simulink model "main_damaged_aircraft"  (R2025b)
settings: Solver=ode45  StartTime=0.0  StopTime=10  RelTol=1e-3
InitFcn:
  | init_project;
undefined symbols (not defined in the file): P, theta_d
libraries: aerolibprivatev1p5 x2, aerolibatmos2 x1, aerolibobsolete x1
settings Model: Creator=22149  LastModifiedBy=22149
settings DataIOCC: SaveFormat=StructureWithTime

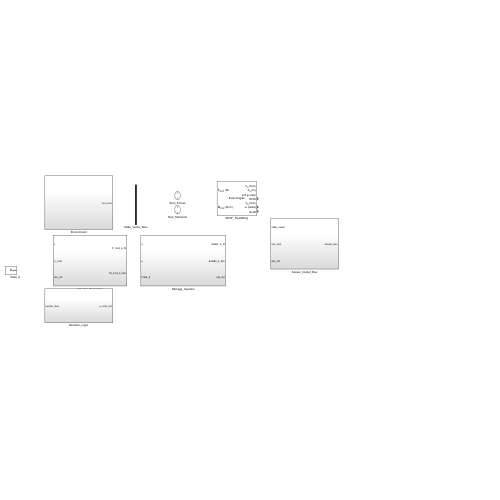
[thumbnail: Simulink's stored preview of the top-level diagram]
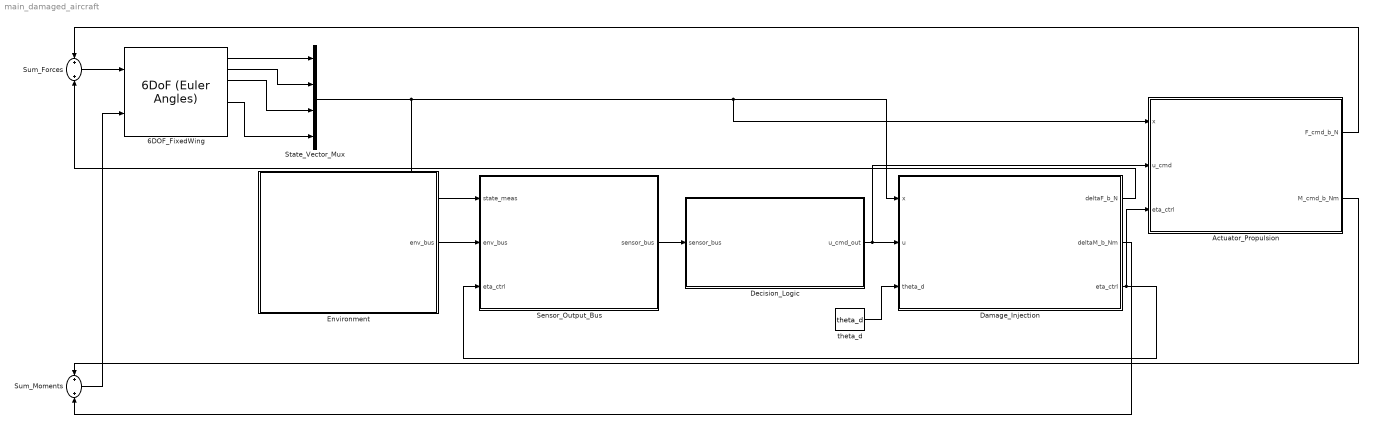
== system main_damaged_aircraft ==
  6DOF_FixedWing : aerolibprivatev1p5/6DoF (Euler Angles)  xme_0=P.initial.pned_m'  Vm_0=P.initial.uvw_mps'  eul_0=P.initial.euler_rad'  pm_0=P.initial.pqr_rps'  Mass=P.aircraft.mass  Inertia=P.aircraft.inertia
  Actuator_Propulsion : Subsystem
  Damage_Injection : Subsystem
  Decision_Logic : Subsystem
  Environment : Subsystem
  Sensor_Output_Bus : Subsystem
  State_Vector_Mux : Mux
  Sum_Forces : Sum
  Sum_Moments : Sum
  theta_d : Constant  Value=theta_d
  wires:
  Sum_Forces/1 -> 6DOF_FixedWing/1
  Sensor_Output_Bus/1(sensor_bus) -> Decision_Logic/1(sensor_bus)
  6DOF_FixedWing/2 -> State_Vector_Mux/2
  Sum_Moments/1 -> 6DOF_FixedWing/2
  theta_d/1 -> Damage_Injection/3(theta_d)
  6DOF_FixedWing/1 -> State_Vector_Mux/1
  6DOF_FixedWing/3 -> State_Vector_Mux/3
  State_Vector_Mux/1 -> Actuator_Propulsion/1(x), Damage_Injection/1(x), Sensor_Output_Bus/1(state_meas)
  Environment/1(env_bus) -> Sensor_Output_Bus/2(env_bus)
  6DOF_FixedWing/5 -> State_Vector_Mux/4
  Decision_Logic/1(u_cmd_out) -> Actuator_Propulsion/2(u_cmd), Damage_Injection/2(u)
  Damage_Injection/1(deltaF_b_N) -> Sum_Forces/2
  Damage_Injection/2(deltaM_b_Nm) -> Sum_Moments/2
  Damage_Injection/3(eta_ctrl) -> Sensor_Output_Bus/3(eta_ctrl), Actuator_Propulsion/3(eta_ctrl)
  Actuator_Propulsion/1(F_cmd_b_N) -> Sum_Forces/1
  Actuator_Propulsion/2(M_cmd_b_Nm) -> Sum_Moments/1

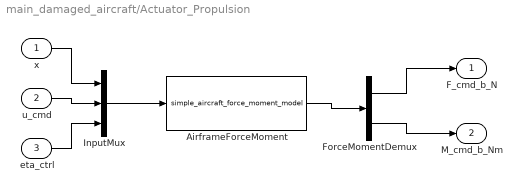
== system main_damaged_aircraft/Actuator_Propulsion ==
  x : Inport
  u_cmd : Inport  Port=2
  eta_ctrl : Inport  Port=3
  AirframeForceMoment : MATLABFcn  MATLABFcn=simple_aircraft_force_moment_model  OutputDimensions=6
  ForceMomentDemux : Demux  Outputs=[3 3]
  InputMux : Mux  Inputs=3
  F_cmd_b_N : Outport
  M_cmd_b_Nm : Outport  Port=2
  wires:
  x/1 -> InputMux/1
  u_cmd/1 -> InputMux/2
  eta_ctrl/1 -> InputMux/3
  InputMux/1 -> AirframeForceMoment/1
  AirframeForceMoment/1 -> ForceMomentDemux/1
  ForceMomentDemux/1 -> F_cmd_b_N/1
  ForceMomentDemux/2 -> M_cmd_b_Nm/1

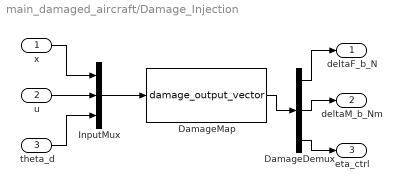
== system main_damaged_aircraft/Damage_Injection ==
  x : Inport
  u : Inport  Port=2
  theta_d : Inport  Port=3
  DamageDemux : Demux  Outputs=[3 3 4]
  DamageMap : MATLABFcn  MATLABFcn=damage_output_vector  OutputDimensions=10
  InputMux : Mux  Inputs=3
  deltaF_b_N : Outport
  deltaM_b_Nm : Outport  Port=2
  eta_ctrl : Outport  Port=3
  wires:
  x/1 -> InputMux/1
  u/1 -> InputMux/2
  theta_d/1 -> InputMux/3
  InputMux/1 -> DamageMap/1
  DamageMap/1 -> DamageDemux/1
  DamageDemux/1 -> deltaF_b_N/1
  DamageDemux/2 -> deltaM_b_Nm/1
  DamageDemux/3 -> eta_ctrl/1

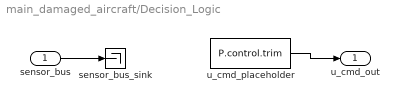
== system main_damaged_aircraft/Decision_Logic ==
  sensor_bus : Inport
  sensor_bus_sink : Terminator
  u_cmd_placeholder : Constant  Value=P.control.trim
  u_cmd_out : Outport
  wires:
  sensor_bus/1 -> sensor_bus_sink/1
  u_cmd_placeholder/1 -> u_cmd_out/1

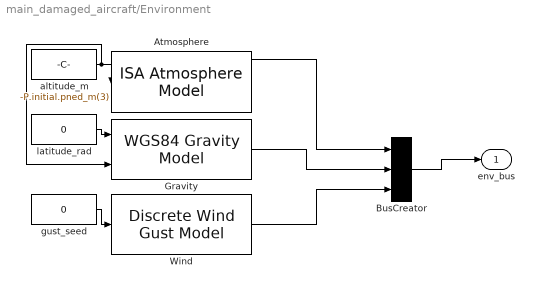
== system main_damaged_aircraft/Environment ==
  Atmosphere : aerolibatmos2/ISA Atmosphere Model  useExtended=off  action=None  custom=off  viscosityOut=off  g=9.80665  gamma=1.4  R=287.0531  L=0.0065  h_trop=11000  h_strat=20000  rho0=1.225  P0=101325  T0=288.15  h0=0  S=110.4  Tref=273.15  muref=1.716e-5
  BusCreator : BusCreator  Inputs=3
  Gravity : aerolibobsolete/WGS84 Gravity Model  model=WGS84 Taylor Series  units=Metric (MKS)  no_atmos=on  precessing=on  month=February  day=1  year=2000  no_centrifugal=on  action=Warning
  Wind : aerolibprivatev1p5/Discrete Wind Gust Model  v_units=meters/second  Gx=on  Gy=on  Gz=on  t_0=5  d_m=[120 120 80]  v_m=[3.5 3.5 3.0]
  altitude_m : Constant  Value=-P.initial.pned_m(3)
  gust_seed : Constant  Value=0
  latitude_rad : Constant  Value=0
  env_bus : Outport
  wires:
  altitude_m/1 -> Atmosphere/1, Gravity/2
  latitude_rad/1 -> Gravity/1
  gust_seed/1 -> Wind/1
  Atmosphere/1 -> BusCreator/1
  Gravity/1 -> BusCreator/2
  Wind/1 -> BusCreator/3
  BusCreator/1 -> env_bus/1

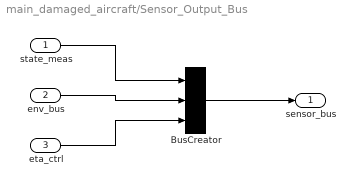
== system main_damaged_aircraft/Sensor_Output_Bus ==
  state_meas : Inport
  env_bus : Inport  Port=2
  eta_ctrl : Inport  Port=3
  BusCreator : BusCreator  Inputs=3
  sensor_bus : Outport
  wires:
  state_meas/1 -> BusCreator/1
  env_bus/1 -> BusCreator/2
  eta_ctrl/1 -> BusCreator/3
  BusCreator/1 -> sensor_bus/1
